simulink model "trialwithoutLMS2receivers"  (R2018a)
settings: Solver=VariableStepAuto  StartTime=0.0  StopTime=10.0  RelTol=1e-3
undefined symbols (not defined in the file or in its folder): doppler
libraries: commutil2 x4, commchan3 x2, commdigbbndpm3 x2, dspxfrm3 x2, dspindex x2, commmimo x2, commseqgen2 x1, commrandsrc2 x1, commsink2 x1, dspobslib x1
settings Model: Creator=commlab7  LastModifiedBy=Varshini Rajesh
settings DataIOCC: ReturnWorkspaceOutputs=on
settings SFSimCC: SimUseLocalCustomCode=on
settings RTWCC: RTWUseLocalCustomCode=on

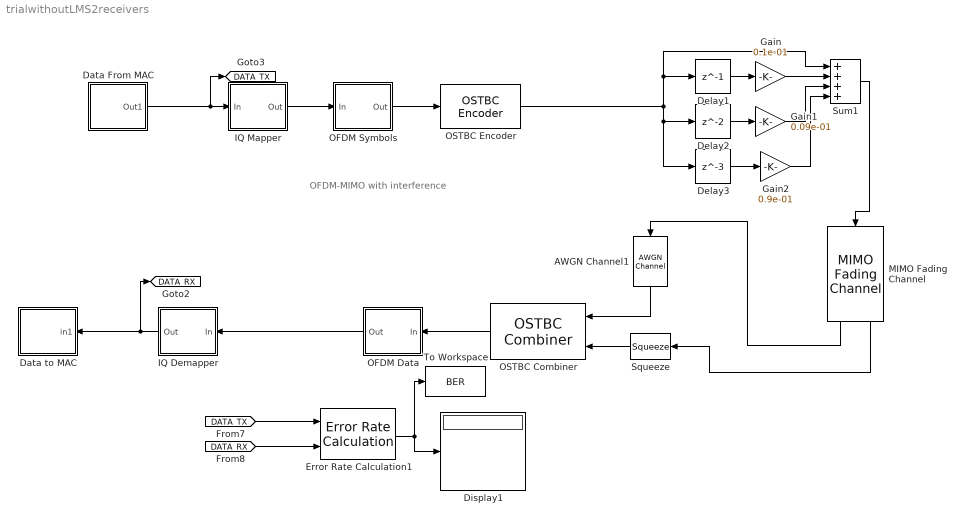
== system trialwithoutLMS2receivers ==
  note: OFDM-MIMO with interference
  AWGN Channel1 : commchan3/AWGN Channel  InputProcessing=Columns as channels (frame based)  seed=67  noiseMode="Signal to noise ratio  (SNR)"  EbNodB=10  EsNodB=10  SNRdB=10  bitsPerSym=1  Ps=1  Tsym=1  variance=1
  Data From MAC : Subsystem
      mask Display: disp('Data Source');
  Data to MAC : Subsystem
      mask Display: disp('Data Sink');
  Delay1 : Delay  DelayLength=1  InputProcessing=Columns as channels (frame based)
  Delay2 : Delay  InputProcessing=Columns as channels (frame based)
  Delay3 : Delay  DelayLength=3  InputProcessing=Columns as channels (frame based)
  Display1 : Display
  Error Rate Calculation1 : commsink2/Error Rate Calculation  N=0  st_delay=0  cp_mode=Entire frame  subframe=[]  PMode=Port  WsName=ErrorVec  RsMode2=off  stop=on  numErr=1e3  maxBits=1e6
  Gain : Gain  Gain=0.1e-01
  Gain1 : Gain  Gain=0.09e-01
  Gain2 : Gain  Gain=0.9e-01
  IQ Demapper : Subsystem
      mask Display: disp('IQ Demapper');
  IQ Mapper : Subsystem
      mask Display: disp('IQ Mapper');
  MIMO Fading Channel : commchan3/MIMO Fading Channel  InheritSampleRate=on  SampleRate=-1  PathDelays=0  AveragePathGains=0  NormalizePathGains=on  FadingDistribution=Rayleigh  KFactor=3  DirectPathDopplerShift=0  DirectPathInitialPhase=0  MaximumDopplerShift=0.001  DopplerSpectrum=doppler( 'Jakes' )  SpatialCorrelationSpecification=None  SpatialCorrelationMatrix=[1 0 0 0; 0 1 0 0; 0 0 1 0; 0 0 0 1]  NumTransmitAntennas=4  NumReceiveAntennas=2  TransmitCorrelationMatrix=[1 0; 0 1]  ReceiveCorrelationMatrix=[1 0; 0 1]  AntennaSelection=Off  NormalizeChannelOutputs=on  SimulateUsing=Interpreted execution  FadingTechnique=Filtered Gaussian noise  NumSinusoids=48  InitialTimeSource=Property  InitialTime=0  ChannelInterpolationMethod=Polyphase  RandomStream=mt19937ar with seed  Seed=73  PathGainsOutputPort=on  Visualization=Off  AntennaPairsToDisplay=[ 1, 1 ]  PathsForDopplerDisplay=1  SamplesToDisplay=25%
      settings: SourceProductName=Communications System Toolbox  SourceProductBaseCode=CM
  OFDM Data : Subsystem
      mask Display: disp('OFDM \n Demodulator');
  OFDM Symbols : Subsystem
      mask Display: disp(' OFDM \n Modulation');
  OSTBC Combiner : commmimo/OSTBC Combiner  numTx=4  rate=1/2  numRx=2  roundingMode=Floor  overflowMode=Wrap  OvFlMode=off  OvFlModeLastStrValue=off  crossProductWordLen=32  crossProductFracLen=16  crossSumWordLen=32  crossSumFracLen=16  egyProductWordLen=32  egyProductFracLen=16  egySumWordLen=32  egySumFracLen=16  divisionWordLen=32  divisionFracLen=16  divisionDataTypeStr=Inherit: Same as accumulator  divisionLastDataTypeStr=Inherit: Same as accumulator
      settings: SourceProductName=Communications System Toolbox  SourceProductBaseCode=CM
  OSTBC Encoder : commmimo/OSTBC Encoder  numTx=4  rate=1/2  overflowMode=Wrap  OvFlMode=off  OvFlModeLastStrValue=off
      settings: SourceProductName=Communications System Toolbox  SourceProductBaseCode=CM
  Squeeze : Squeeze
  Sum1 : Sum  Inputs=++++  SaturateOnIntegerOverflow=on
  To Workspace : ToWorkspace  VariableName=BER  SampleTime=-1
      settings: MaxDataPoints=1
  tag scope: DATA_RX=global, DATA_TX=global
  wires:
  Data From MAC/1(Out1) -> IQ Mapper/1(In), [DATA_TX]
  IQ Mapper/1(Out) -> OFDM Symbols/1(In)
  [DATA_RX] -> Error Rate Calculation1/2
  IQ Demapper/1(Out) -> Data to MAC/1(in1), [DATA_RX]
  [DATA_TX] -> Error Rate Calculation1/1
  Error Rate Calculation1/1 -> To Workspace/1, Display1/1
  OFDM Symbols/1(Out) -> OSTBC Encoder/1
  MIMO Fading Channel/1 -> AWGN Channel1/1
  AWGN Channel1/1 -> OSTBC Combiner/1
  Squeeze/1 -> OSTBC Combiner/2
  MIMO Fading Channel/2 -> Squeeze/1
  Delay1/1 -> Gain/1
  OSTBC Encoder/1 -> Sum1/1, Delay1/1, Delay3/1, Delay2/1
  Delay2/1 -> Gain1/1
  Gain1/1 -> Sum1/3
  Gain2/1 -> Sum1/4
  Delay3/1 -> Gain2/1
  Gain/1 -> Sum1/2
  Sum1/1 -> MIMO Fading Channel/1
  OSTBC Combiner/1 -> OFDM Data/1(In)
  OFDM Data/1(Out) -> IQ Demapper/1(In)

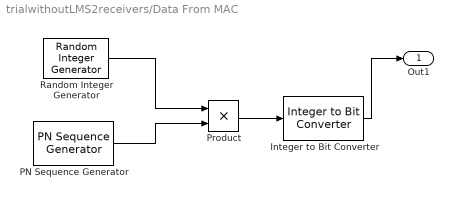
== system trialwithoutLMS2receivers/Data From MAC ==
  Integer to Bit Converter : commutil2/Integer to Bit Converter  nbits=2  signedInputValues=Unsigned  bitOrder=MSB first  outDtype=Inherit via internal rule
  PN Sequence Generator : commseqgen2/PN Sequence Generator  poly=[1 0 0 0 0 1 1]  ini_sta=[1 0 0 1 0 0]  outBitMaskSource=Dialog parameter  shift=0  outVarSiz=off  maxOutSizeMode=Dialog parameter  maxOutSize=[10 1]  Ts=1/192  frameBased=off  sampPerFrame=1  reset=off  bitPackedOutputs=off  outDataType=double  numPackedBits=8  bitPackDataSigned=off  bitPackedOutDType=double
      settings: SourceProductName=Communications System Toolbox  SourceProductBaseCode=CM
  Product : Product  RndMeth=Zero
  Random Integer Generator : commrandsrc2/Random Integer Generator  mul=2  seed=37  Ts=1/192  frameBased=on  sampPerFrame=192  orient=off  outDataType=double
      settings: SourceProductName=Communications System Toolbox  SourceProductBaseCode=CM
  Out1 : Outport  VectorParamsAs1DForOutWhenUnconnected=on
  wires:
  Product/1 -> Integer to Bit Converter/1
  Random Integer Generator/1 -> Product/1
  PN Sequence Generator/1 -> Product/2
  Integer to Bit Converter/1 -> Out1/1

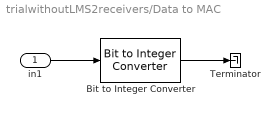
== system trialwithoutLMS2receivers/Data to MAC ==
  in1 : Inport
  Bit to Integer Converter : commutil2/Bit to Integer Converter  nbits=2  bitOrder=MSB first  signedOutputValues=Unsigned  outDtype=Same as input  outDtypeSigned=Inherit via internal rule
  Terminator : Terminator
  wires:
  in1/1 -> Bit to Integer Converter/1
  Bit to Integer Converter/1 -> Terminator/1

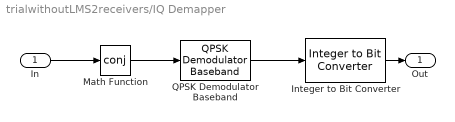
== system trialwithoutLMS2receivers/IQ Demapper ==
  In : Inport
  Integer to Bit Converter : commutil2/Integer to Bit Converter  nbits=2  signedInputValues=Unsigned  bitOrder=MSB first  outDtype=Same as input
  Math Function : Math  Operator=conj  SaturateOnIntegerOverflow=on
  QPSK Demodulator Baseband : commdigbbndpm3/QPSK Demodulator Baseband  OutType=Integer  DecType=Hard decision  VarSource=Dialog  Variance=1  Dec=Gray  Ph=pi/4  outDtype1=Inherit via internal rule  outDtype2=Inherit via internal rule  derotateFactorWordLen=16  derotateFactorDataTypeStr=Inherit: Same word length as input  derotateFactorLastDataTypeStr=Inherit: Same word length as input
  Out : Outport  VectorParamsAs1DForOutWhenUnconnected=on
  wires:
  QPSK Demodulator Baseband/1 -> Integer to Bit Converter/1
  In/1 -> Math Function/1
  Math Function/1 -> QPSK Demodulator Baseband/1
  Integer to Bit Converter/1 -> Out/1

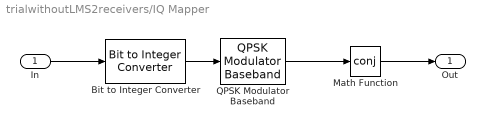
== system trialwithoutLMS2receivers/IQ Mapper ==
  In : Inport
  Bit to Integer Converter : commutil2/Bit to Integer Converter  nbits=2  bitOrder=MSB first  signedOutputValues=Unsigned  outDtype=Same as input  outDtypeSigned=Inherit via internal rule
  Math Function : Math  Operator=conj  SaturateOnIntegerOverflow=on
  QPSK Modulator Baseband : commdigbbndpm3/QPSK Modulator Baseband  InType=Integer  Enc=Gray  Ph=pi/4  outDtype=double  outWordLen=16  outUDDataType=sfix(16)  outFracLenMode=Best precision  outFracLen=15  outDataTypeStr=double  outLastDataTypeStr=double
  Out : Outport  VectorParamsAs1DForOutWhenUnconnected=on
  wires:
  In/1 -> Bit to Integer Converter/1
  Math Function/1 -> Out/1
  Bit to Integer Converter/1 -> QPSK Modulator Baseband/1
  QPSK Modulator Baseband/1 -> Math Function/1

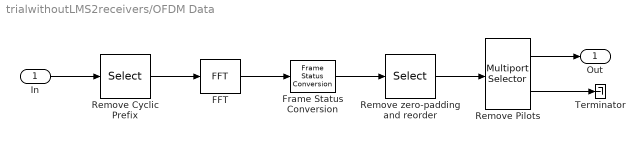
== system trialwithoutLMS2receivers/OFDM Data ==
  In : Inport
  FFT : dspxfrm3/FFT  FFTImplementation=Auto  CompMethod=Table lookup  TableOpt=HYBRID  TableOptActive=Speed  BitRevOrder=off  Normalize=off  InheritFFTLength=on  FFTLength=64  WrapInput=on  roundingMode=Floor  overflowMode=off  firstCoeffDataTypeStr=Inherit: Same word length as input  firstCoeffLastDataTypeStr=Inherit: Same word length as input  outputMin=[]  outputMax=[]
  Frame Status Conversion : dspobslib/Frame Status Conversion  growRefPort=off  outframe=Frame-based
      settings: SourceProductName=DSP System Toolbox  SourceProductBaseCode=DS
  Remove zero-padding and reorder : Selector  InputPortWidth=256  IndexOptions=Index vector (dialog)  Indices=[29:128 130:229]  OutputSizes=1
  Remove Pilots : dspindex/Multiport Selector  rowsOrCols=Rows  idxCellArray={[1:12 14:37 39:62 64:87 89:112 114:137 139:162 164:187 189:200],[13 38 63 88 113 138 163 188]}  idxErrMode=Clip Index
  Remove Cyclic Prefix : Selector  NumberOfDimensions=2  InputPortWidth=320  IndexOptions=Index vector (dialog),Index vector (dialog)  Indices=[65:320],1  OutputSizes=1,1
  Terminator : Terminator
  Out : Outport  VectorParamsAs1DForOutWhenUnconnected=on
  wires:
  Frame Status Conversion/1 -> Remove zero-padding and reorder/1
  FFT/1 -> Frame Status Conversion/1
  In/1 -> Remove Cyclic Prefix/1
  Remove zero-padding and reorder/1 -> Remove Pilots/1
  Remove Pilots/1 -> Out/1
  Remove Pilots/2 -> Terminator/1
  Remove Cyclic Prefix/1 -> FFT/1

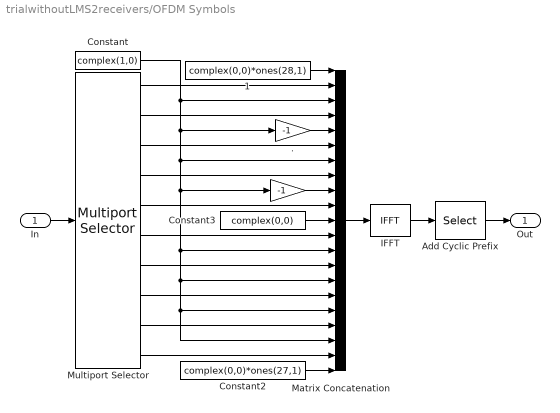
== system trialwithoutLMS2receivers/OFDM Symbols ==
  In : Inport
  " " : Gain  Gain=-1
  " 1" : Constant  Value=complex(0,0)*ones(28,1)
  . : Gain  Gain=-1
  Add Cyclic Prefix : Selector  InputPortWidth=256  IndexOptions=Index vector (dialog)  Indices=[193:256 1:256]  OutputSizes=1
  Constant : Constant  Value=complex(1,0)
  Constant2 : Constant  Value=complex(0,0)*ones(27,1)
  Constant3 : Constant  Value=complex(0,0)
  IFFT : dspxfrm3/IFFT  FFTImplementation=Auto  CompMethod=Table lookup  TableOpt=HYBRID  TableOptActive=Speed  BitRevOrder=off  cs_in=off  Normalize=on  InheritFFTLength=on  FFTLength=64  WrapInput=on  mode=Complex  outSamplingMode=Frame based  roundingMode=Floor  overflowMode=off  firstCoeffDataTypeStr=Inherit: Same word length as input  firstCoeffLastDataTypeStr=Inherit: Same word length as input  outputMin=[]  outputMax=[]
      settings: SourceProductName=DSP System Toolbox
  Matrix Concatenation : Concatenate  NumInputs=21  Mode=Multidimensional array
  Multiport Selector : dspindex/Multiport Selector  rowsOrCols=Rows  idxCellArray={1:12, 13:36, 37:60, 61:84, 85:96, 97:108, 109:132, 133:156, 157:180, 181:192}  idxErrMode=Clip Index
  Out : Outport  VectorParamsAs1DForOutWhenUnconnected=on
  wires:
  In/1 -> Multiport Selector/1
  Multiport Selector/9 -> Matrix Concatenation/18
  Multiport Selector/8 -> Matrix Concatenation/16
  Multiport Selector/7 -> Matrix Concatenation/14
  Multiport Selector/6 -> Matrix Concatenation/12
  Multiport Selector/5 -> Matrix Concatenation/10
  Multiport Selector/4 -> Matrix Concatenation/8
  Multiport Selector/3 -> Matrix Concatenation/6
  Multiport Selector/2 -> Matrix Concatenation/4
  Multiport Selector/1 -> Matrix Concatenation/2
  Multiport Selector/10 -> Matrix Concatenation/20
  Constant/1 -> Matrix Concatenation/3, Matrix Concatenation/7, " "/1, Matrix Concatenation/13, Matrix Concatenation/15, Matrix Concatenation/19, Matrix Concatenation/17, ./1
  " 1"/1 -> Matrix Concatenation/1
  Constant2/1 -> Matrix Concatenation/21
  ./1 -> Matrix Concatenation/5
  " "/1 -> Matrix Concatenation/9
  Constant3/1 -> Matrix Concatenation/11
  IFFT/1 -> Add Cyclic Prefix/1
  Matrix Concatenation/1 -> IFFT/1
  Add Cyclic Prefix/1 -> Out/1
